simulink model "DCMotorLoopwBacklashAngle"  (R2015a)
settings: Solver=ode45  StartTime=0.0  StopTime=60  RelTol=1e-10  AbsTol=1e-10
values from neighbouring files (symbols this model uses):
  c = 0.001    [CSD_HW_1_Script.m]    (also in Plotshit.m)
  d = 5*pi/180    (= 0.0872664625997)    [CSD_HW_1_Script.m]    (also in Plotshit.m)
  Jl = 0.02    [CSD_HW_1_Script.m]    (also in Plotshit.m)
  Jm = 0.001    [CSD_HW_1_Script.m]    (also in Plotshit.m)
  K = [0.1 30]    [CSD_HW_1_Script.m]    (also in Plotshit.m)
  Kt = 0.03    [CSD_HW_1_Script.m]    (also in Plotshit.m)
  N = 3    [CSD_HW_1_Script.m]    (also in Plotshit.m)
  R = 0.1    [CSD_HW_1_Script.m]    (also in Plotshit.m)
undefined symbols (not defined in the file or in its folder): ii
libraries: cstblocks x1
settings Model: Creator=yarde_000  LastModifiedBy=yarde_000

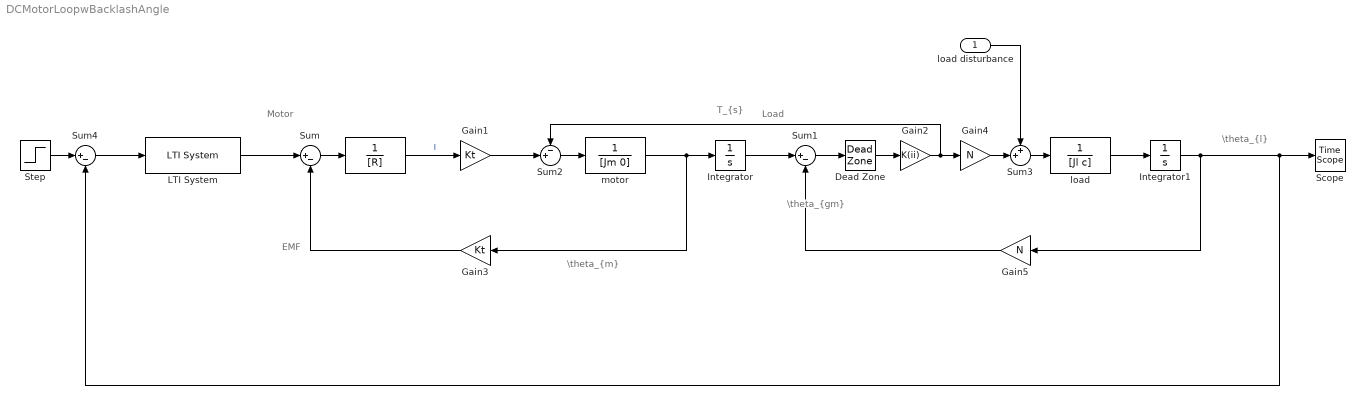
== system DCMotorLoopwBacklashAngle ==
  note: Load
  note: Motor
  note: \theta_{m}
  note: EMF
  note: T_{s}
  note: \theta_{l}
  note: \theta_{gm}
  load disturbance : Inport
  " " : TransferFcn  Denominator=[R]
  " load" : TransferFcn  Denominator=[Jl c]
  " motor" : TransferFcn  Denominator=[Jm 0]
  Dead Zone : DeadZone  LowerValue=-d/2  UpperValue=d/2  SaturateOnIntegerOverflow=on
  Gain1 : Gain  Gain=Kt
      mask Display: disp('K_t','texmode','on')
  Gain2 : Gain  Gain=K(ii)
      mask Display: disp('K','texmode','on')
  Gain3 : Gain  Gain=Kt
      mask Display: disp('K_t','texmode','on')
  Gain4 : Gain  Gain=N
      mask Display: disp('N','texmode','on')
  Gain5 : Gain  Gain=N
      mask Display: disp('N','texmode','on')
  Integrator : Integrator
  Integrator1 : Integrator
  LTI System : cstblocks/LTI System  sys=C  IC=[]
  Scope : TimeScope
  Step : Step  Time=0  After=pi/6  SampleTime=0
  Sum : Sum  Inputs=|+-
  Sum1 : Sum  Inputs=|+-
  Sum2 : Sum  Inputs=-+|
  Sum3 : Sum  Inputs=++|
  Sum4 : Sum  Inputs=|+-
  wires:
  Sum/1 -> " "/1
  " "/1 -> Gain1/1  "I"
  " motor"/1 -> Gain3/1, Integrator/1
  Gain3/1 -> Sum/2
  Integrator/1 -> Sum1/1
  Sum1/1 -> Dead Zone/1
  Dead Zone/1 -> Gain2/1
  Gain1/1 -> Sum2/2
  Sum2/1 -> " motor"/1
  " load"/1 -> Integrator1/1
  Integrator1/1 -> Gain5/1, Sum4/2, Scope/1
  Gain5/1 -> Sum1/2
  LTI System/1 -> Sum/1
  Gain4/1 -> Sum3/2
  Sum3/1 -> " load"/1
  load disturbance/1 -> Sum3/1
  Gain2/1 -> Sum2/1, Gain4/1
  Sum4/1 -> LTI System/1
  Step/1 -> Sum4/1
